simulink model "modelo_sistema_original"  (Simulink 7.5)
settings: Solver=ode45  StartTime=0.0  StopTime=100  RelTol=1e-3
libraries: simulink_need_slupdate x1
settings Model: Creator=manu  LastModifiedBy=manu

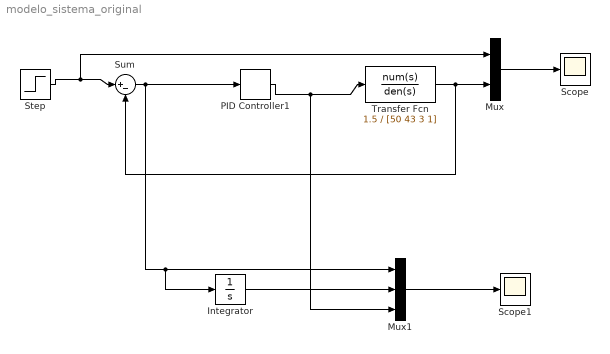
== system modelo_sistema_original ==
  Integrator : Integrator
  Mux : Mux  Inputs=2
  Mux1 : Mux  Inputs=3
  PID Controller1 : simulink_need_slupdate/PID Controller  SystemSampleTime=-1  P=6.36  I=0.4968  D=20.3561
  Scope : Scope
      settings: TimeRange=100  YMin=0  YMax=1.4
  Scope1 : Scope
      settings: TimeRange=100  YMin=0  YMax=1.4
  Step : Step  Time=0  SampleTime=0.01
  Sum : Sum  Inputs=|+-  OutDataType=sfix(16)  OutScaling=2^0  SaturateOnIntegerOverflow=on  InputSameDT=on  OutDataTypeStr=Inherit: Same as first input
  Transfer Fcn : TransferFcn  Numerator=1.5  Denominator=[50 43 3 1]
  wires:
  PID Controller1/1 -> Transfer Fcn/1, Mux1/3
  Sum/1 -> PID Controller1/1, Mux1/1, Integrator/1
  Step/1 -> Sum/1, Mux/1
  Mux/1 -> Scope/1
  Transfer Fcn/1 -> Mux/2, Sum/2
  Mux1/1 -> Scope1/1
  Integrator/1 -> Mux1/2
